simulink model "sampleModel1950"  (R2023a)
settings: Solver=VariableStepAuto  StartTime=0.0  StopTime=10.0  RelTol=1e-3
libraries: hdlsllib x10
settings Model: Creator=user1  LastModifiedBy=user1

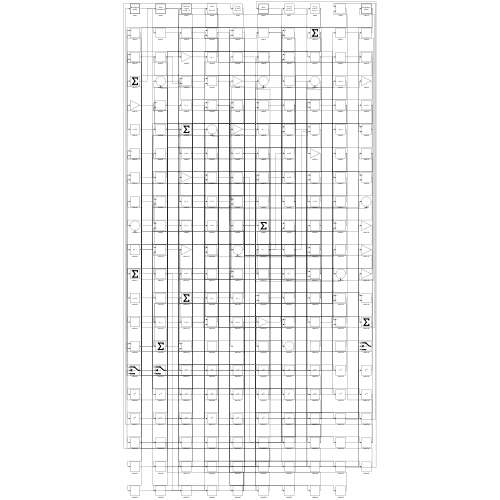
[thumbnail: Simulink's stored preview of the top-level diagram]
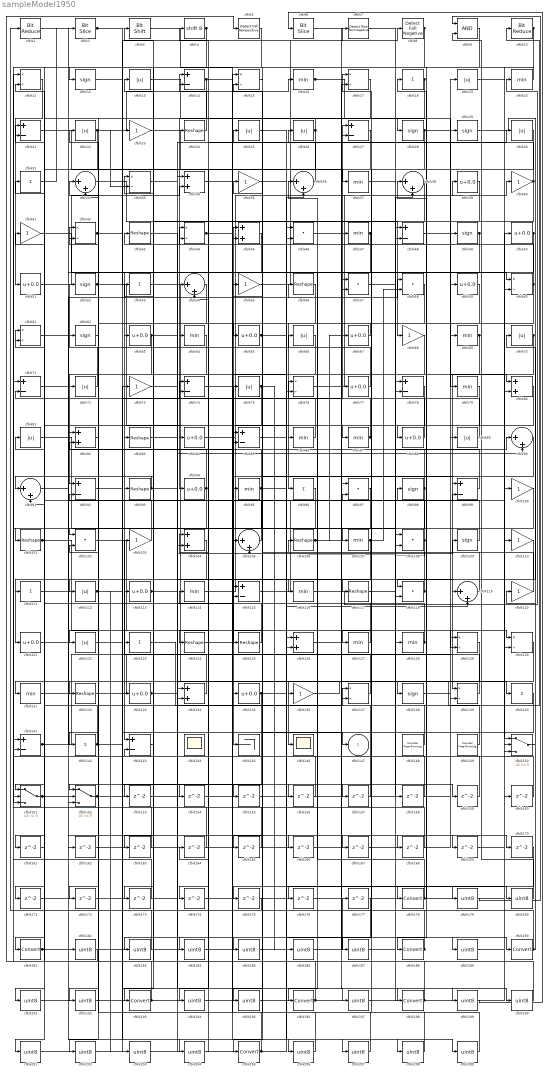
== system sampleModel1950 ==
  cfblk1 : hdlsllib/Logic and Bit Operations/Bit Reduce  mode=AND
  cfblk10 : hdlsllib/Logic and Bit Operations/Bit Reduce  mode=AND
  cfblk{23,35,40..41,55,68,73,100,103,110,120,136} (12 alike) : Gain
  cfblk{24,43,56,83,93,101,106,117,124..125,132} (11 alike) : Reshape
  cfblk{46,57..58,97,102,108,118} (7 alike) : DotProduct  OutDataTypeStr=Inherit: Inherit via internal rule
  cfblk{34,45,80,82,104,126,134} (7 alike) : Sum
  cfblk{32,36,38,54,90..91,105,119} (8 alike) : Sum  Inputs=|++
  cfblk{16,20,37,47,64,69,79,86..87,95,107,114,116,127..128,131} (16 alike) : MinMax
  cfblk{12,28..29,49,52,62,98,109,138} (9 alike) : Signum
  cfblk{11,15,17,33,42,44,60..61,76,129..130,137,139} (13 alike) : Product  Inputs=*/  RndMeth=Zero  SaturateOnIntegerOverflow=on
  cfblk{18,31,53,96,111,123,140,142} (8 alike) : Sum  Inputs=+
  cfblk{13,19,22,25..26,30,66,70,72,75,81,89,112,122} (14 alike) : Abs  SaturateOnIntegerOverflow=off
  cfblk{39,50..51,59,63,65,67,77,84,88,94,113,121,133,135} (15 alike) : Bias  Bias=0.0  SaturateOnIntegerOverflow=off
  cfblk{14,21,27,48,71,74,78,85,92,99,115,141,143} (13 alike) : Sum  Inputs=+-
  cfblk144 : Scope
      settings: Floating=on
  cfblk145 : Terminator
  cfblk146 : Scope
  cfblk148 : hdlsllib/Sources/Counter Free-Running  NumBits=16  tsamp=-1
  cfblk149 : hdlsllib/Sources/Counter Free-Running  NumBits=16  tsamp=-1
  cfblk150 : Switch  SaturateOnIntegerOverflow=off  InputSameDT=off
  cfblk151 : Switch  SaturateOnIntegerOverflow=off  InputSameDT=off
  cfblk152 : Switch  SaturateOnIntegerOverflow=off  InputSameDT=off
  cfblk{153..177} (25 alike) : Delay  SampleTime=1
  cfblk{178,181,188,190,193,196,198,205} (8 alike) : DataTypeConversion  SaturateOnIntegerOverflow=off  RndMeth=Floor
  cfblk{179..180,182..187,189,191..192,194..195,197,199..204,206..209} (24 alike) : DataTypeConversion  OutDataTypeStr=uint8  SaturateOnIntegerOverflow=off  RndMeth=Floor
  cfblk2 : hdlsllib/Logic and Bit Operations/Bit Slice  lidx=7  ridx=0
  cfblk3 : hdlsllib/Logic and Bit Operations/Bit Shift  mode=Shift Left Logical  N=0
  cfblk4 : ArithShift  BitShiftNumber=8
  cfblk5 : hdlsllib/Logic and Bit Operations/Detect Fall Nonpositive  vinit=0  OutDataTypeStr=boolean
  cfblk6 : hdlsllib/Logic and Bit Operations/Bit Slice  lidx=7  ridx=0
  cfblk7 : hdlsllib/Logic and Bit Operations/Detect Rise Nonnegative  vinit=0  OutDataTypeStr=boolean
  cfblk8 : hdlsllib/Logic and Bit Operations/Detect Fall Negative  vinit=0  OutDataTypeStr=boolean
  cfblk9 : Logic  AllPortsSameDT=off  OutDataTypeStr=boolean
  cfblk147 : Outport  VectorParamsAs1DForOutWhenUnconnected=off
  wires:
  cfblk152/1 -> cfblk89/1, cfblk159/1
  cfblk76/1 -> cfblk40/1
  cfblk81/1 -> cfblk107/1
  cfblk55/1 -> cfblk7/1
  cfblk40/1 -> cfblk26/1, cfblk175/1
  cfblk29/1 -> cfblk118/1
  cfblk6/1 -> cfblk198/1
  cfblk96/1 -> cfblk101/1
  cfblk102/1 -> cfblk130/1
  cfblk15/1 -> cfblk205/1
  cfblk24/1 -> cfblk14/1
  cfblk63/1 -> cfblk92/1, cfblk108/2
  cfblk116/1 -> cfblk20/1
  cfblk26/1 -> cfblk122/1, cfblk24/1
  cfblk47/1 -> cfblk143/1, cfblk173/1
  cfblk123/1 -> cfblk137/1
  cfblk37/1 -> cfblk60/1
  cfblk30/1 -> cfblk127/1
  cfblk56/1 -> cfblk96/1
  cfblk53/1 -> cfblk146/1
  cfblk17/1 -> cfblk94/1
  cfblk134/1 -> cfblk103/1
  cfblk74/1 -> cfblk145/1
  cfblk107/1 -> cfblk121/1, cfblk58/2
  cfblk87/1 -> cfblk27/1, cfblk117/1
  cfblk62/1 -> cfblk102/1
  cfblk143/1 -> cfblk13/1
  cfblk110/1 -> cfblk188/1
  cfblk109/1 -> cfblk18/1
  cfblk70/1 -> cfblk139/1, cfblk176/1
  cfblk115/1 -> cfblk50/1
  cfblk151/1 -> cfblk166/1, cfblk167/1
  cfblk93/1 -> cfblk91/1, cfblk90/2
  cfblk20/1 -> cfblk12/1
  cfblk11/1 -> cfblk51/1
  cfblk136/1 -> cfblk10/1
  cfblk114/1 -> cfblk39/1
  cfblk9/1 -> cfblk178/1
  cfblk120/1 -> cfblk92/2
  cfblk138/1 -> cfblk29/1
  cfblk95/1 -> cfblk77/1, cfblk129/2, cfblk141/2, cfblk33/1
  cfblk127/1 -> cfblk45/1
  cfblk31/1 -> cfblk2/1
  cfblk13/1 -> cfblk28/1
  cfblk139/1 -> cfblk44/1
  cfblk100/1 -> cfblk196/1
  cfblk23/1 -> cfblk37/1
  cfblk119/1 -> cfblk43/1
  cfblk65/1 -> cfblk119/2, cfblk189/1
  cfblk4/1 -> cfblk83/1, cfblk93/1
  cfblk51/1 -> cfblk34/2
  cfblk150/1 -> cfblk70/1
  cfblk86/1 -> cfblk61/1
  cfblk125/1 -> cfblk113/1
  cfblk129/1 -> cfblk131/1
  cfblk148/1 -> cfblk114/1
  cfblk32/1 -> cfblk68/1
  cfblk79/1 -> cfblk88/1
  cfblk124/1 -> cfblk45/2
  cfblk117/1 -> cfblk90/1
  cfblk132/1 -> cfblk69/1
  cfblk75/1 -> cfblk171/1, cfblk186/1
  cfblk141/1 -> cfblk19/1, cfblk99/2
  cfblk8/1 -> cfblk137/2, cfblk151/3
  cfblk133/1 -> cfblk109/1, cfblk138/1
  cfblk99/1 -> cfblk17/1
  cfblk52/1 -> cfblk84/1, cfblk8/1
  cfblk84/1 -> cfblk86/1
  cfblk131/1 -> cfblk59/1
  cfblk5/1 -> cfblk181/1
  cfblk1/1 -> cfblk72/1
  cfblk18/1 -> cfblk151/1, cfblk112/1
  cfblk149/1 -> cfblk32/1
  cfblk112/1 -> cfblk76/1, cfblk203/1
  cfblk22/1 -> cfblk16/1, cfblk33/2, cfblk201/1
  cfblk71/1 -> cfblk58/1
  cfblk126/1 -> cfblk190/1
  cfblk2/1 -> cfblk23/1, cfblk168/1
  cfblk33/1 -> cfblk30/1
  cfblk21/1 -> cfblk95/1
  cfblk44/1 -> cfblk76/2, cfblk206/1
  cfblk58/1 -> cfblk82/1
  cfblk42/1 -> cfblk22/1, cfblk154/1
  cfblk27/1 -> cfblk124/1
  cfblk60/1 -> cfblk25/1, cfblk116/1
  cfblk90/1 -> cfblk125/1
  cfblk106/1 -> cfblk130/2, cfblk67/1
  cfblk105/1 -> cfblk14/2
  cfblk10/1 -> cfblk60/2, cfblk85/1
  cfblk101/1 -> cfblk135/1, cfblk85/2
  cfblk72/1 -> cfblk52/1
  cfblk19/1 -> cfblk150/1
  cfblk137/1 -> cfblk106/1
  cfblk91/1 -> cfblk56/1
  cfblk28/1 -> cfblk80/1, cfblk87/1
  cfblk41/1 -> cfblk128/1
  cfblk49/1 -> cfblk142/1, cfblk174/1
  cfblk67/1 -> cfblk65/1
  cfblk82/1 -> cfblk132/1
  cfblk78/1 -> cfblk193/1
  cfblk16/1 -> cfblk49/1, cfblk180/1
  cfblk3/1 -> cfblk75/1
  cfblk88/1 -> cfblk21/1
  cfblk48/1 -> cfblk79/1
  cfblk14/1 -> cfblk152/1, cfblk199/1
  cfblk98/1 -> cfblk74/1, cfblk111/1
  cfblk108/1 -> cfblk71/2, cfblk105/1, cfblk105/2
  cfblk36/1 -> cfblk4/1
  cfblk57/1 -> cfblk118/2
  cfblk46/1 -> cfblk47/1
  cfblk89/1 -> cfblk74/2
  cfblk142/1 -> cfblk81/1, cfblk147/1
  cfblk39/1 -> cfblk63/1
  cfblk43/1 -> cfblk140/1
  cfblk135/1 -> cfblk169/1, cfblk192/1
  cfblk45/1 -> cfblk64/1
  cfblk50/1 -> cfblk136/1, cfblk152/2
  cfblk113/1 -> cfblk3/1, cfblk119/1, cfblk115/2
  cfblk103/1 -> cfblk11/2
  cfblk77/1 -> cfblk53/1
  cfblk128/1 -> cfblk104/1, cfblk31/1
  cfblk94/1 -> cfblk42/1, cfblk104/2
  cfblk38/1 -> cfblk48/2
  cfblk69/1 -> cfblk152/3, cfblk187/1
  cfblk34/1 -> cfblk99/1
  cfblk118/1 -> cfblk62/1, cfblk55/1
  cfblk59/1 -> cfblk153/1
  cfblk153/1 -> cfblk129/1
  cfblk130/1 -> cfblk155/1
  cfblk155/1 -> cfblk48/1
  cfblk83/1 -> cfblk156/1
  cfblk156/1 -> cfblk143/2
  cfblk92/1 -> cfblk157/1
  cfblk157/1 -> cfblk44/2
  cfblk7/1 -> cfblk158/1
  cfblk158/1 -> cfblk61/2
  cfblk159/1 -> cfblk71/1
  cfblk160/1 -> cfblk38/1
  cfblk104/1 -> cfblk161/1
  cfblk111/1 -> cfblk162/1
  cfblk162/1 -> cfblk17/2
  cfblk66/1 -> cfblk163/1
  cfblk163/1 -> cfblk11/1
  cfblk164/1 -> cfblk21/2
  cfblk140/1 -> cfblk165/1
  cfblk165/1 -> cfblk91/2
  cfblk166/1 -> cfblk36/1
  cfblk167/1 -> cfblk139/2
  cfblk168/1 -> cfblk42/2
  cfblk169/1 -> cfblk80/2
  cfblk85/1 -> cfblk170/1
  cfblk171/1 -> cfblk134/2
  cfblk64/1 -> cfblk172/1
  cfblk172/1 -> cfblk34/1
  cfblk173/1 -> cfblk141/1
  cfblk174/1 -> cfblk150/2
  cfblk175/1 -> cfblk1/1
  cfblk176/1 -> cfblk150/3
  cfblk178/1 -> cfblk66/1, cfblk98/1
  cfblk25/1 -> cfblk179/1
  cfblk179/1 -> cfblk9/1
  cfblk180/1 -> cfblk9/2
  cfblk181/1 -> cfblk133/1, cfblk38/2
  cfblk61/1 -> cfblk182/1
  cfblk182/1 -> cfblk5/1
  cfblk177/1 -> cfblk183/1
  cfblk183/1 -> cfblk32/2
  cfblk68/1 -> cfblk184/1
  cfblk184/1 -> cfblk177/1
  cfblk97/1 -> cfblk185/1
  cfblk185/1 -> cfblk57/2
  cfblk186/1 -> cfblk97/1
  cfblk187/1 -> cfblk97/2
  cfblk188/1 -> cfblk164/1, cfblk57/1
  cfblk189/1 -> cfblk110/1
  cfblk190/1 -> cfblk108/1, cfblk120/1
  cfblk161/1 -> cfblk191/1
  cfblk191/1 -> cfblk126/1
  cfblk192/1 -> cfblk126/2
  cfblk193/1 -> cfblk36/2, cfblk102/2
  cfblk80/1 -> cfblk194/1
  cfblk194/1 -> cfblk78/1
  cfblk170/1 -> cfblk195/1
  cfblk195/1 -> cfblk78/2
  cfblk196/1 -> cfblk151/2, cfblk123/1
  cfblk12/1 -> cfblk197/1
  cfblk197/1 -> cfblk100/1
  cfblk198/1 -> cfblk160/1, cfblk41/1
  cfblk199/1 -> cfblk6/1
  cfblk73/1 -> cfblk200/1
  cfblk200/1 -> cfblk46/1
  cfblk201/1 -> cfblk73/1
  cfblk54/1 -> cfblk202/1
  cfblk202/1 -> cfblk46/2
  cfblk203/1 -> cfblk54/1
  cfblk121/1 -> cfblk204/1
  cfblk204/1 -> cfblk54/2
  cfblk205/1 -> cfblk115/1, cfblk82/2, cfblk134/1
  cfblk206/1 -> cfblk15/1
  cfblk154/1 -> cfblk207/1
  cfblk207/1 -> cfblk15/2
  cfblk35/1 -> cfblk208/1
  cfblk208/1 -> cfblk27/2
  cfblk122/1 -> cfblk209/1
  cfblk209/1 -> cfblk35/1
